simulink model "Linear_SS_model_validation"  (R2019b)
settings: Solver=VariableStepAuto  StartTime=0.0  StopTime=10.0  RelTol=1e-3
values from neighbouring files (symbols this model uses):
  A = [-(Cf+Cr)/(m*Vx), -1-(lf*Cf-lr*Cr)/(m*Vx^2) ... (first row only)    [LQI_for_LateralStability_LinMod_slipNDyaw.m]    (also in LQR.m; LQR_Model_Initialization.m; LQR_Simulink_testData_DLC.mat = [-4.40211640212  -0.830687830688; 20.8695652174  -5.18678260; LQR_test_data_DLC.mat = [-4.40211640212  -0.830687830688; 20.8695652174  -5.18678260)
  B = [Cf/(m*Vx);(lf*Cf)/Iz]    [LQI_for_LateralStability_LinMod_slipNDyaw.m]    (also in LQR.m; LQR_Model_Initialization.m; LQR_Simulink_testData_DLC.mat = [1.60846560847 15.8608695652]; LQR_test_data_DLC.mat = [1.60846560847 15.8608695652])
settings Model: Creator=Shouvik Chakraborty  LastModifiedBy=Shouvik Chakraborty
settings SFSimCC: CustomCodeUndefinedFunction=UseInterfaceOnly

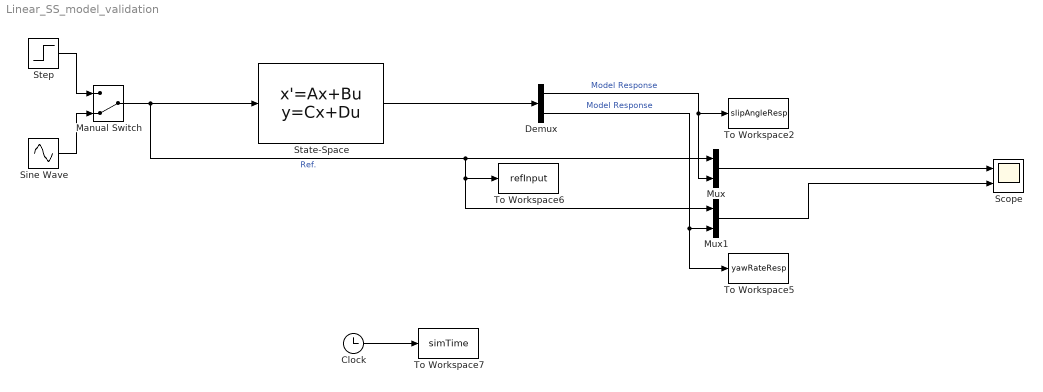
== system Linear_SS_model_validation ==
  Clock : Clock
  Demux : Demux  Outputs=2
  Manual Switch : ManualSwitch  CurrentSetting=0
  Mux : Mux  Inputs=2
  Mux1 : Mux  Inputs=2
  Scope : Scope  NumInputPorts=2
  Sine Wave : Sin  Amplitude=2  Frequency=0.5  SampleTime=0
  State-Space : StateSpace  A=A  B=B  C=eye(2,2)  D=[0;0]  InitialCondition=0
  Step : Step  SampleTime=0
  To Workspace2 : ToWorkspace  VariableName=slipAngleResp  SampleTime=-1
  To Workspace5 : ToWorkspace  VariableName=yawRateResp  SampleTime=-1
  To Workspace6 : ToWorkspace  VariableName=refInput  SampleTime=-1
  To Workspace7 : ToWorkspace  VariableName=simTime  SampleTime=-1
  wires:
  Mux/1 -> Scope/1
  State-Space/1 -> Demux/1
  Step/1 -> Manual Switch/1
  Mux1/1 -> Scope/2
  Demux/2 -> To Workspace5/1, Mux1/2  "Model Response"
  Manual Switch/1 -> To Workspace6/1, Mux1/1, Mux/1, State-Space/1  "Ref."
  Demux/1 -> To Workspace2/1, Mux/2  "Model Response"
  Clock/1 -> To Workspace7/1
  Sine Wave/1 -> Manual Switch/2
